simulink subsystem "acc_nom"  (R2025b)
settings: Solver=VariableStepAuto  StartTime=0.0  StopTime=10.0  RelTol=1e-3
settings Model: Creator=sanborkl  LastModifiedBy=sanborkl

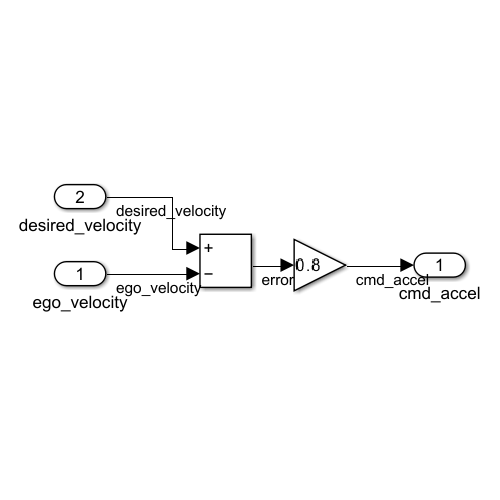
[thumbnail: Simulink's stored preview of the top-level diagram]
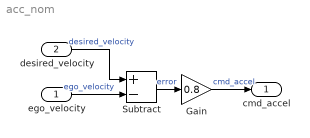
== system acc_nom ==
  ego_velocity : Inport
  desired_velocity : Inport  Port=2
  Gain : Gain  Gain=0.8
  Subtract : Sum  Inputs=+-
  cmd_accel : Outport
  wires:
  Gain/1 -> cmd_accel/1  "cmd_accel"
  desired_velocity/1 -> Subtract/1  "desired_velocity"
  Subtract/1 -> Gain/1  "error"
  ego_velocity/1 -> Subtract/2  "ego_velocity"
